simulink model "Model_6DOF"  (R2022a)
settings: Solver=FixedStepAuto  StartTime=0.0  StopTime=Tf  FixedStep=0.05  RelTol=1e-3
values from neighbouring files (symbols this model uses):
  Ba_0 = [0 0 0 0 0 0]    [run.m]
  Bv_0 = [-5.14444 0 0 0 0 0]    [run.m]
  Bx_0 = [0 0 -20 0 0 0]    [run.m]
  psi_ref = 0    [run.m]
  Seastate = 0    [run.m]
  Tf = 5000    [run.m]
  v_ref = Bv_0(1)    [run.m]
  z_ref = Bx_0(3)    [run.m]
undefined symbols (not defined in the file or in its folder): Bb, Cp, Cp_prime, dA_BP1, dA_BP2, dA_Hull, dA_PH, dA_Sail, dA_SProot, dA_X1a, dA_X1b, dA_X2a, dA_X2b, dA_X3a, dA_X3b, dA_X4a, dA_X4b, Ixx, Ixy, Ixz, Iyy, Iyz, Izz, Mb, n_BP1, n_BP2, n_Hull, n_PH, n_Sail, n_SProot, n_X2a, n_X2b, n_X3a, n_X4a, n_X4b, nt_BP1, nt_BP2, nt_Hull, nt_PH, nt_Sail, nt_SProot, nt_X1a, nt_X1b, nt_X2a, nt_X2b, nt_X3a, nt_X3b, nt_X4a, nt_X4b, tknots, vt1_BP1, vt1_BP2, vt1_Hull, vt1_PH, vt1_Sail, vt1_SProot, vt1_X1a, vt1_X1b, vt1_X2a, vt1_X2b ... (+39)
libraries: simulink x8
(part 3 of 5)

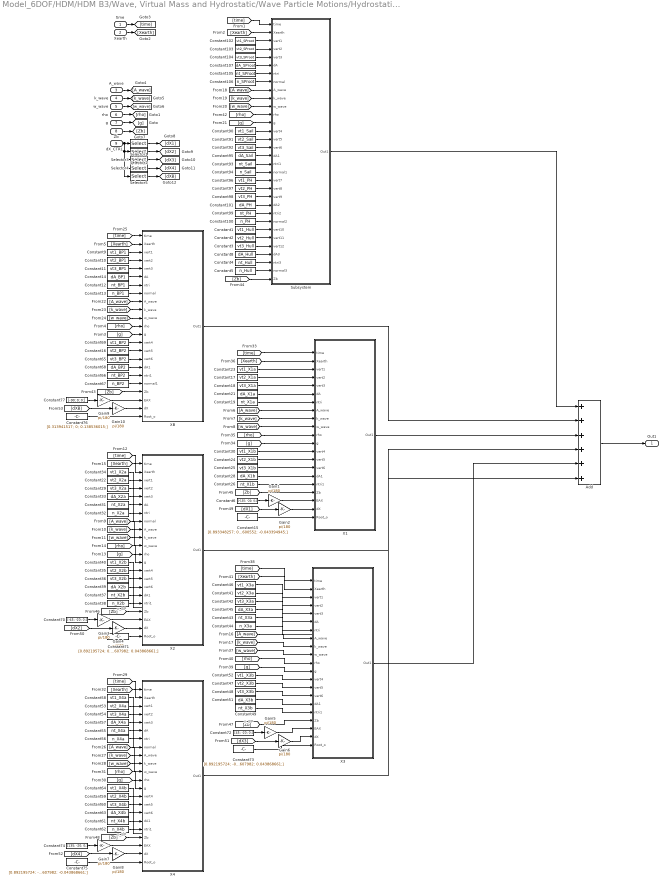
== system Model_6DOF/HDM/HDM B3/Wave, Virtual Mass and Hydrostatic/Wave Particle Motions/Hydrostatic Forces and Moments ==
  note: n_BP
  note: n_BP
  note: n_BP
  time : Inport
  Xearth : Inport  Port=2
  A_wave : Inport  Port=3
  k_wave : Inport  Port=4
  w_wave : Inport  Port=5
  rho : Inport  Port=6
  g : Inport  Port=7
  Zb : Inport  Port=8
  dX_CTRL : Inport  Port=9
  Add : Sum  Inputs=6
  Constant1 : Constant  Value=vt1_Hull
  Constant10 : Constant  Value=vt2_BP1
  Constant100 : Constant  Value=n_PH
  Constant101 : Constant  Value=dA_PH
  Constant102 : Constant  Value=vt1_SProot
  Constant103 : Constant  Value=vt2_SProot
  Constant104 : Constant  Value=vt3_SProot
  Constant105 : Constant  Value=nt_SProot
  Constant106 : Constant  Value=n_SProot
  Constant107 : Constant  Value=dA_SProot
  Constant11 : Constant  Value=vt3_BP1
  Constant12 : Constant  Value=nt_BP1
  Constant13 : Constant  Value=n_BP1
  Constant14 : Constant  Value=dA_BP1
  Constant15 : Constant  Value=|
      | [0.893348257;
      | 0.043600552;
      | -0.043394945;]
  Constant16 : Constant  Value=vt2_BP2
  Constant17 : Constant  Value=vt2_X1a
  Constant18 : Constant  Value=vt3_X1a
  Constant19 : Constant  Value=nt_X1a
  Constant2 : Constant  Value=vt2_Hull
  Constant21 : Constant  Value=dA_X1a
  Constant22 : Constant  Value=vt2_X2a
  Constant23 : Constant  Value=vt1_X1a
  Constant24 : Constant  Value=vt2_X1b
  Constant25 : Constant  Value=vt3_X1b
  Constant26 : Constant  Value=nt_X1b
  Constant28 : Constant  Value=dA_X1b
  Constant29 : Constant  Value=vt3_X2a
  Constant3 : Constant  Value=vt3_Hull
  Constant30 : Constant  Value=vt1_X1b
  Constant31 : Constant  Value=nt_X2a
  Constant32 : Constant  Value=n_X2a
  Constant33 : Constant  Value=dA_X2a
  Constant34 : Constant  Value=vt1_X2a
  Constant35 : Constant  Value=vt2_X2b
  Constant36 : Constant  Value=vt3_X2b
  Constant37 : Constant  Value=nt_X2b
  Constant38 : Constant  Value=n_X2b
  Constant39 : Constant  Value=dA_X2b
  Constant4 : Constant  Value=nt_Hull
  Constant40 : Constant  Value=vt1_X2b
  Constant41 : Constant  Value=vt2_X3a
  Constant42 : Constant  Value=vt3_X3a
  Constant43 : Constant  Value=nt_X3a
  Constant44 : Constant  Value=n_X3a
  Constant45 : Constant  Value=dA_X3a
  Constant46 : Constant  Value=vt1_X3a
  Constant47 : Constant  Value=vt2_X3b
  Constant48 : Constant  Value=vt3_X3b
  Constant49 : Constant  Value=nt_X3b
  Constant5 : Constant  Value=n_Hull
  Constant51 : Constant  Value=dA_X3b
  Constant52 : Constant  Value=vt1_X3b
  Constant53 : Constant  Value=vt2_X4a
  Constant54 : Constant  Value=vt3_X4a
  Constant55 : Constant  Value=nt_X4a
  Constant56 : Constant  Value=n_X4a
  Constant57 : Constant  Value=dA_X4a
  Constant58 : Constant  Value=vt1_X4a
  Constant59 : Constant  Value=vt2_X4b
  Constant6 : Constant  Value=[-135; -20; 0;]
  Constant60 : Constant  Value=vt3_X4b
  Constant61 : Constant  Value=nt_X4b
  Constant62 : Constant  Value=n_X4b
  Constant63 : Constant  Value=dA_X4b
  Constant64 : Constant  Value=vt1_X4b
  Constant65 : Constant  Value=vt3_BP2
  Constant66 : Constant  Value=nt_BP2
  Constant67 : Constant  Value=n_BP2
  Constant68 : Constant  Value=dA_BP2
  Constant69 : Constant  Value=vt1_BP2
  Constant70 : Constant  Value=[-45; -20; 0;]
  Constant71 : Constant  Value=|
      | [0.892195724;
      | 0.043607982;
      | 0.043868661;]
  Constant72 : Constant  Value=[45; -20; 0;]
  Constant73 : Constant  Value=|
      | [0.892195724;
      | -0.043607982;
      | 0.043868661;]
  Constant74 : Constant  Value=[135; -20; 0;]
  Constant75 : Constant  Value=|
      | [0.892195724;
      | -0.043607982;
      | -0.043868661;]
  Constant76 : Constant  Value=|
      | [0.313941517;
      | 0;
      | 0.138536015;]
  Constant77 : Constant  Value=[-90; 0; 0;]
  Constant8 : Constant  Value=dA_Hull
  Constant9 : Constant  Value=vt1_BP1
  Constant90 : Constant  Value=vt1_Sail
  Constant91 : Constant  Value=vt2_Sail
  Constant92 : Constant  Value=vt3_Sail
  Constant93 : Constant  Value=nt_Sail
  Constant94 : Constant  Value=n_Sail
  Constant95 : Constant  Value=dA_Sail
  Constant96 : Constant  Value=vt1_PH
  Constant97 : Constant  Value=vt2_PH
  Constant98 : Constant  Value=vt3_PH
  Constant99 : Constant  Value=nt_PH
  Gain{1..10} (10 alike) : Gain  Gain=pi/180
  Selector1 : Selector  InputPortWidth=5  IndexOptions=Index vector (dialog)  Indices=1  OutputSizes=1
  Selector2 : Selector  InputPortWidth=5  IndexOptions=Index vector (dialog)  Indices=2  OutputSizes=1
  Selector3 : Selector  InputPortWidth=5  IndexOptions=Index vector (dialog)  Indices=3  OutputSizes=1
  Selector4 : Selector  InputPortWidth=5  IndexOptions=Index vector (dialog)  Indices=4  OutputSizes=1
  Selector5 : Selector  InputPortWidth=5  IndexOptions=Index vector (dialog)  Indices=5  OutputSizes=1
  Subsystem : Subsystem
  X1 : Subsystem
  X2 : Subsystem
  X3 : Subsystem
  X4 : Subsystem
  XB : Subsystem
  Out1 : Outport
  wires:
  time/1 -> [time]
  Xearth/1 -> [Xearth]
  A_wave/1 -> [A_wave]
  k_wave/1 -> [k_wave]
  w_wave/1 -> [w_wave]
  rho/1 -> [rho]
  g/1 -> [g]
  Constant94/1 -> Subsystem/19(normal1)
  Constant61/1 -> X4/18(ntri1)
  Constant57/1 -> X4/6(dA)
  [Zb] -> X4/19(Zb)
  [Zb] -> X3/18(Zb)
  Constant101/1 -> Subsystem/23(dA2)
  Constant16/1 -> XB/15(vert5)
  [Zb] -> X1/18(Zb)
  [Zb] -> X2/19(Zb)
  Constant98/1 -> Subsystem/22(vert9)
  Constant99/1 -> Subsystem/24(ntri2)
  Constant37/1 -> X2/18(ntri1)
  [Zb] -> XB/20(Zb)
  [time] -> X3/1(time)
  [Xearth] -> X1/2(Xearth)
  [w_wave] -> Subsystem/11(w_wave)
  Constant93/1 -> Subsystem/18(ntri1)
  [g] -> X2/13(g)
  Constant28/1 -> X1/16(dA1)
  [w_wave] -> X3/10(w_wave)
  Constant8/1 -> Subsystem/29(dA3)
  Constant95/1 -> Subsystem/17(dA1)
  [A_wave] -> X4/9(A_wave)
  Constant33/1 -> X2/6(dA)
  [rho] -> X4/12(rho)
  [time] -> Subsystem/1(time)
  Constant48/1 -> X3/15(vert6)
  [rho] -> Subsystem/12(rho)
  Constant60/1 -> X4/16(vert6)
  [k_wave] -> Subsystem/10(k_wave)
  Constant19/1 -> X1/7(ntri)
  [g] -> Subsystem/13(g)
  Constant102/1 -> Subsystem/3(vert1)
  Constant106/1 -> Subsystem/8(normal)
  [Xearth] -> Subsystem/2(Xearth)
  Constant107/1 -> Subsystem/6(dA)
  Constant105/1 -> Subsystem/7(ntri)
  [g] -> X4/13(g)
  Constant11/1 -> XB/5(vert3)
  Constant34/1 -> X2/3(vert1)
  Constant63/1 -> X4/17(dA1)
  [A_wave] -> X1/8(A_wave)
  Constant41/1 -> X3/4(vert2)
  [k_wave] -> X2/10(k_wave)
  Constant22/1 -> X2/4(vert2)
  Constant49/1 -> X3/17(ntri1)
  [Xearth] -> XB/2(Xearth)
  [rho] -> X2/12(rho)
  [rho] -> X3/11(rho)
  Constant55/1 -> X4/7(ntri)
  Constant45/1 -> X3/6(dA)
  Constant40/1 -> X2/14(vert4)
  Constant18/1 -> X1/5(vert3)
  [g] -> X1/12(g)
  Constant35/1 -> X2/15(vert5)
  Constant39/1 -> X2/17(dA1)
  Constant32/1 -> X2/8(normal)
  Constant47/1 -> X3/14(vert5)
  [w_wave] -> X4/11(w_wave)
  Constant44/1 -> ?
  [k_wave] -> X1/9(k_wave)
  Constant53/1 -> X4/4(vert2)
  [w_wave] -> XB/11(w_wave)
  [Xearth] -> X2/2(Xearth)
  [time] -> XB/1(time)
  [rho] -> XB/12(rho)
  Constant4/1 -> Subsystem/30(ntri3)
  Constant59/1 -> X4/15(vert5)
  Constant51/1 -> X3/16(dA1)
  Constant52/1 -> X3/13(vert4)
  Constant14/1 -> XB/6(dA)
  [Xearth] -> X3/2(Xearth)
  Constant25/1 -> X1/15(vert6)
  Constant67/1 -> XB/19(normal1)
  [Zb] -> Subsystem/32(Zb)
  Constant65/1 -> XB/16(vert6)
  Constant104/1 -> Subsystem/5(vert3)
  Constant13/1 -> XB/8(normal)
  Constant69/1 -> XB/14(vert4)
  Constant43/1 -> X3/7(ntri)
  [k_wave] -> X3/9(k_wave)
  [A_wave] -> X2/9(A_wave)
  Constant17/1 -> X1/4(vert2)
  [k_wave] -> XB/10(k_wave)
  Constant68/1 -> XB/17(dA1)
  Constant46/1 -> X3/3(vert1)
  Constant23/1 -> X1/3(vert1)
  Constant9/1 -> XB/3(vert1)
  Constant62/1 -> ?
  [A_wave] -> XB/9(A_wave)
  Constant26/1 -> X1/17(ntri1)
  Constant56/1 -> X4/8(normal)
  Constant24/1 -> X1/14(vert5)
  Constant12/1 -> XB/7(ntri)
  [g] -> X3/12(g)
  [w_wave] -> X1/10(w_wave)
  Constant100/1 -> Subsystem/25(normal2)
  Constant92/1 -> Subsystem/16(vert6)
  Constant30/1 -> X1/13(vert4)
  [time] -> X2/1(time)
  [rho] -> X1/11(rho)
  Constant91/1 -> Subsystem/15(vert5)
  [time] -> X1/1(time)
  Constant1/1 -> Subsystem/26(vert10)
  Constant31/1 -> X2/7(ntri)
  [w_wave] -> X2/11(w_wave)
  Constant21/1 -> X1/6(dA)
  Constant90/1 -> Subsystem/14(vert4)
  Constant96/1 -> Subsystem/20(vert7)
  Constant36/1 -> X2/16(vert6)
  Constant29/1 -> X2/5(vert3)
  [Xearth] -> X4/2(Xearth)
  Constant64/1 -> X4/14(vert4)
  Constant97/1 -> Subsystem/21(vert8)
  Constant2/1 -> Subsystem/27(vert11)
  Constant66/1 -> XB/18(ntri1)
  Constant54/1 -> X4/5(vert3)
  Constant38/1 -> ?
  [k_wave] -> X4/10(k_wave)
  [time] -> X4/1(time)
  Constant10/1 -> XB/4(vert2)
  [A_wave] -> Subsystem/9(A_wave)
  Add/1 -> Out1/1
  Constant103/1 -> Subsystem/4(vert2)
  Constant3/1 -> Subsystem/28(vert12)
  [g] -> XB/13(g)
  Constant42/1 -> X3/5(vert3)
  Constant58/1 -> X4/3(vert1)
  Constant5/1 -> Subsystem/31(normal3)
  [A_wave] -> X3/8(A_wave)
  Zb/1 -> [Zb]
  Constant6/1 -> Gain1/1
  Gain1/1 -> X1/19(EAX)
  dX_CTRL/1 -> Selector2/1, Selector3/1, Selector5/1, Selector4/1, Selector1/1
  Selector1/1 -> [dX1]
  Selector2/1 -> [dX2]
  Selector3/1 -> [dX3]
  Selector4/1 -> [dX4]
  Selector5/1 -> [dXB]
  [dX1] -> Gain2/1
  Gain2/1 -> X1/20(dX)
  Constant15/1 -> X1/21(Root_o)
  Constant70/1 -> Gain3/1
  Gain3/1 -> X2/20(EAX)
  [dX2] -> Gain4/1
  Gain4/1 -> X2/21(dX)
  Constant71/1 -> X2/22(Root_o)
  Gain5/1 -> X3/19(EAX)
  [dX3] -> Gain6/1
  Constant72/1 -> Gain5/1
  Gain6/1 -> X3/20(dX)
  Constant73/1 -> X3/21(Root_o)
  Constant75/1 -> X4/22(Root_o)
  Gain7/1 -> X4/20(EAX)
  Constant74/1 -> Gain7/1
  [dX4] -> Gain8/1
  Gain8/1 -> X4/21(dX)
  Constant77/1 -> Gain9/1
  Gain9/1 -> XB/21(EAX)
  [dXB] -> Gain10/1
  Constant76/1 -> XB/23(Root_o)
  Gain10/1 -> XB/22(dX)
  X4/1(Out1) -> Add/6
  X3/1(Out1) -> Add/5
  X2/1(Out1) -> Add/4
  X1/1(Out1) -> Add/3
  XB/1(Out1) -> Add/2
  Subsystem/1(Out1) -> Add/1

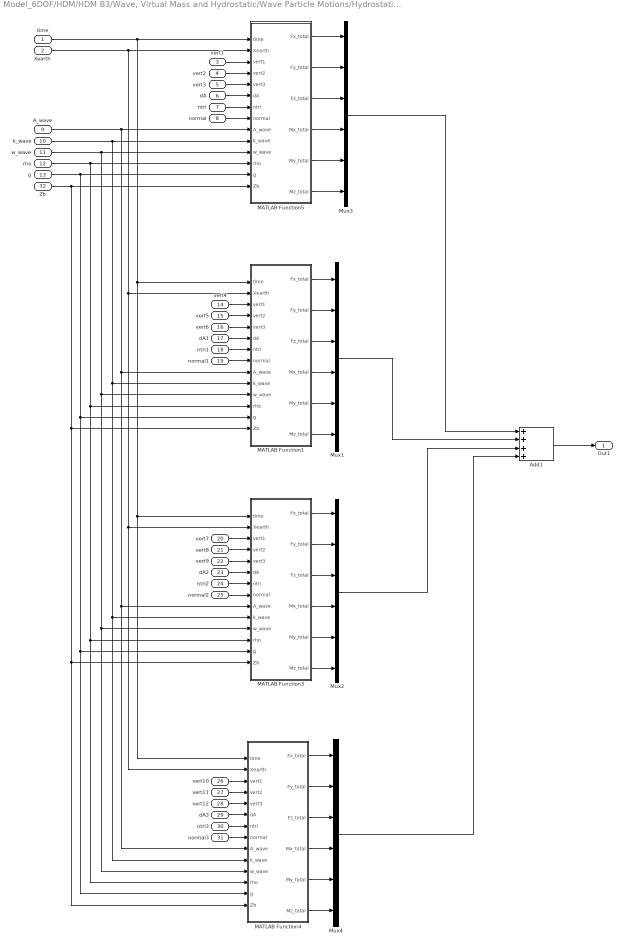
== system Model_6DOF/HDM/HDM B3/Wave, Virtual Mass and Hydrostatic/Wave Particle Motions/Hydrostatic Forces and Moments/Subsystem ==
  time : Inport
  Xearth : Inport  Port=2
  vert1 : Inport  Port=3
  vert2 : Inport  Port=4
  vert3 : Inport  Port=5
  dA : Inport  Port=6
  ntri : Inport  Port=7
  normal : Inport  Port=8
  A_wave : Inport  Port=9
  k_wave : Inport  Port=10
  w_wave : Inport  Port=11
  rho : Inport  Port=12
  g : Inport  Port=13
  vert4 : Inport  Port=14
  vert5 : Inport  Port=15
  vert6 : Inport  Port=16
  dA1 : Inport  Port=17
  ntri1 : Inport  Port=18
  normal1 : Inport  Port=19
  vert7 : Inport  Port=20
  vert8 : Inport  Port=21
  vert9 : Inport  Port=22
  dA2 : Inport  Port=23
  ntri2 : Inport  Port=24
  normal2 : Inport  Port=25
  vert10 : Inport  Port=26
  vert11 : Inport  Port=27
  vert12 : Inport  Port=28
  dA3 : Inport  Port=29
  ntri3 : Inport  Port=30
  normal3 : Inport  Port=31
  Zb : Inport  Port=32
  Add1 : Sum  Inputs=4
  MATLAB Function1 : MATLAB Function  TreatAsAtomicUnit=on
  MATLAB Function3 : MATLAB Function  TreatAsAtomicUnit=on
  MATLAB Function4 : MATLAB Function  TreatAsAtomicUnit=on
  MATLAB Function5 : MATLAB Function  TreatAsAtomicUnit=on
  Mux{1..4} (4 alike) : Mux  Inputs=6
  Out1 : Outport
  wires:
  ntri1/1 -> MATLAB Function1/7(ntri)
  rho/1 -> MATLAB Function5/12(rho), MATLAB Function1/12(rho), MATLAB Function4/12(rho), MATLAB Function3/12(rho)
  vert5/1 -> MATLAB Function1/4(vert2)
  MATLAB Function5/5(My_total) -> Mux3/5
  time/1 -> MATLAB Function5/1(time), MATLAB Function1/1(time), MATLAB Function4/1(time), MATLAB Function3/1(time)
  Xearth/1 -> MATLAB Function5/2(Xearth), MATLAB Function4/2(Xearth), MATLAB Function3/2(Xearth), MATLAB Function1/2(Xearth)
  vert7/1 -> MATLAB Function3/3(vert1)
  MATLAB Function5/4(Mx_total) -> Mux3/4
  Mux3/1 -> Add1/1
  normal1/1 -> MATLAB Function1/8(normal)
  A_wave/1 -> MATLAB Function5/9(A_wave), MATLAB Function1/9(A_wave), MATLAB Function4/9(A_wave), MATLAB Function3/9(A_wave)
  MATLAB Function5/3(Fz_total) -> Mux3/3
  k_wave/1 -> MATLAB Function5/10(k_wave), MATLAB Function1/10(k_wave), MATLAB Function4/10(k_wave), MATLAB Function3/10(k_wave)
  w_wave/1 -> MATLAB Function5/11(w_wave), MATLAB Function1/11(w_wave), MATLAB Function4/11(w_wave), MATLAB Function3/11(w_wave)
  MATLAB Function5/2(Fy_total) -> Mux3/2
  ntri/1 -> MATLAB Function5/7(ntri)
  g/1 -> MATLAB Function5/13(g), MATLAB Function1/13(g), MATLAB Function4/13(g), MATLAB Function3/13(g)
  dA2/1 -> MATLAB Function3/6(dA)
  MATLAB Function5/1(Fx_total) -> Mux3/1
  vert12/1 -> MATLAB Function4/5(vert3)
  normal3/1 -> MATLAB Function4/8(normal)
  vert4/1 -> MATLAB Function1/3(vert1)
  vert9/1 -> MATLAB Function3/5(vert3)
  normal/1 -> MATLAB Function5/8(normal)
  dA/1 -> MATLAB Function5/6(dA)
  MATLAB Function5/6(Mz_total) -> Mux3/6
  vert11/1 -> MATLAB Function4/4(vert2)
  ntri2/1 -> MATLAB Function3/7(ntri)
  ntri3/1 -> MATLAB Function4/7(ntri)
  dA3/1 -> MATLAB Function4/6(dA)
  vert2/1 -> MATLAB Function5/4(vert2)
  Add1/1 -> Out1/1
  vert6/1 -> MATLAB Function1/5(vert3)
  vert3/1 -> MATLAB Function5/5(vert3)
  normal2/1 -> MATLAB Function3/8(normal)
  dA1/1 -> MATLAB Function1/6(dA)
  vert10/1 -> MATLAB Function4/3(vert1)
  vert1/1 -> MATLAB Function5/3(vert1)
  vert8/1 -> MATLAB Function3/4(vert2)
  Zb/1 -> MATLAB Function5/14(Zb), MATLAB Function1/14(Zb), MATLAB Function3/14(Zb), MATLAB Function4/14(Zb)
  Mux2/1 -> Add1/3
  MATLAB Function1/6(Mz_total) -> Mux1/6
  Mux1/1 -> Add1/2
  MATLAB Function1/1(Fx_total) -> Mux1/1
  MATLAB Function1/2(Fy_total) -> Mux1/2
  MATLAB Function1/3(Fz_total) -> Mux1/3
  MATLAB Function1/4(Mx_total) -> Mux1/4
  MATLAB Function1/5(My_total) -> Mux1/5
  MATLAB Function3/5(My_total) -> Mux2/5
  MATLAB Function3/4(Mx_total) -> Mux2/4
  MATLAB Function3/3(Fz_total) -> Mux2/3
  MATLAB Function3/2(Fy_total) -> Mux2/2
  MATLAB Function3/1(Fx_total) -> Mux2/1
  MATLAB Function3/6(Mz_total) -> Mux2/6
  MATLAB Function4/6(Mz_total) -> Mux4/6
  MATLAB Function4/1(Fx_total) -> Mux4/1
  MATLAB Function4/2(Fy_total) -> Mux4/2
  MATLAB Function4/3(Fz_total) -> Mux4/3
  MATLAB Function4/4(Mx_total) -> Mux4/4
  MATLAB Function4/5(My_total) -> Mux4/5
  Mux4/1 -> Add1/4

== system Model_6DOF/HDM/HDM B3/Wave, Virtual Mass and Hydrostatic/Wave Particle Motions/Hydrostatic Forces and Moments/X1 ==
  time : Inport
  Xearth : Inport  Port=2
  vert1 : Inport  Port=3
  vert2 : Inport  Port=4
  vert3 : Inport  Port=5
  dA : Inport  Port=6
  ntri : Inport  Port=7
  A_wave : Inport  Port=8
  k_wave : Inport  Port=9
  w_wave : Inport  Port=10
  rho : Inport  Port=11
  g : Inport  Port=12
  vert4 : Inport  Port=13
  vert5 : Inport  Port=14
  vert6 : Inport  Port=15
  dA1 : Inport  Port=16
  ntri1 : Inport  Port=17
  Zb : Inport  Port=18
  EAX : Inport  Port=19
  dX : Inport  Port=20
  Root_o : Inport  Port=21
  Add1 : Sum
  CG : Constant  Value=[32.3114; 0; 0;]
  MATLAB Function1 : MATLAB Function  TreatAsAtomicUnit=on
  MATLAB Function4 : MATLAB Function  TreatAsAtomicUnit=on
  Mux1 : Mux  Inputs=6
  Mux2 : Mux  Inputs=6
  Out1 : Outport
  wires:
  ntri1/1 -> MATLAB Function1/7(ntri)
  dA1/1 -> MATLAB Function1/6(dA)
  vert6/1 -> MATLAB Function1/5(vert3)
  vert5/1 -> MATLAB Function1/4(vert2)
  vert4/1 -> MATLAB Function1/3(vert1)
  Zb/1 -> MATLAB Function1/13(Zb), MATLAB Function4/13(Zb)
  vert2/1 -> MATLAB Function4/4(vert2)
  ntri/1 -> MATLAB Function4/7(ntri)
  time/1 -> MATLAB Function4/1(time), MATLAB Function1/1(time)
  vert1/1 -> MATLAB Function4/3(vert1)
  Mux1/1 -> Add1/2
  vert3/1 -> MATLAB Function4/5(vert3)
  Mux2/1 -> Add1/1
  MATLAB Function4/2(Fy_total) -> Mux2/2
  MATLAB Function4/6(Mz_total) -> Mux2/6
  g/1 -> MATLAB Function1/12(g), MATLAB Function4/12(g)
  k_wave/1 -> MATLAB Function4/9(k_wave), MATLAB Function1/9(k_wave)
  dA/1 -> MATLAB Function4/6(dA)
  MATLAB Function4/5(My_total) -> Mux2/5
  MATLAB Function1/3(Fz_total) -> Mux1/3
  Add1/1 -> Out1/1
  MATLAB Function1/1(Fx_total) -> Mux1/1
  MATLAB Function4/1(Fx_total) -> Mux2/1
  MATLAB Function1/4(Mx_total) -> Mux1/4
  A_wave/1 -> MATLAB Function1/8(A_wave), MATLAB Function4/8(A_wave)
  rho/1 -> MATLAB Function1/11(rho), MATLAB Function4/11(rho)
  Xearth/1 -> MATLAB Function4/2(Xearth), MATLAB Function1/2(Xearth)
  MATLAB Function1/2(Fy_total) -> Mux1/2
  w_wave/1 -> MATLAB Function1/10(w_wave), MATLAB Function4/10(w_wave)
  MATLAB Function4/4(Mx_total) -> Mux2/4
  MATLAB Function4/3(Fz_total) -> Mux2/3
  EAX/1 -> MATLAB Function1/14(EAX), MATLAB Function4/14(EAX)
  dX/1 -> MATLAB Function4/15(dX), MATLAB Function1/15(dX)
  Root_o/1 -> MATLAB Function1/16(origin), MATLAB Function4/16(origin)
  CG/1 -> MATLAB Function1/17(xcg), MATLAB Function4/17(xcg)
  MATLAB Function1/5(My_total) -> Mux1/5
  MATLAB Function1/6(Mz_total) -> Mux1/6

== system Model_6DOF/HDM/HDM B3/Wave, Virtual Mass and Hydrostatic/Wave Particle Motions/Hydrostatic Forces and Moments/X2 ==
  time : Inport
  Xearth : Inport  Port=2
  vert1 : Inport  Port=3
  vert2 : Inport  Port=4
  vert3 : Inport  Port=5
  dA : Inport  Port=6
  ntri : Inport  Port=7
  normal : Inport  Port=8
  A_wave : Inport  Port=9
  k_wave : Inport  Port=10
  w_wave : Inport  Port=11
  rho : Inport  Port=12
  g : Inport  Port=13
  vert4 : Inport  Port=14
  vert5 : Inport  Port=15
  vert6 : Inport  Port=16
  dA1 : Inport  Port=17
  ntri1 : Inport  Port=18
  Zb : Inport  Port=19
  EAX : Inport  Port=20
  dX : Inport  Port=21
  Root_o : Inport  Port=22
  Add1 : Sum
  CG : Constant  Value=[32.3114; 0; 0;]
  MATLAB Function1 : MATLAB Function  TreatAsAtomicUnit=on
  MATLAB Function4 : MATLAB Function  TreatAsAtomicUnit=on
  Mux1 : Mux  Inputs=6
  Mux2 : Mux  Inputs=6
  Out1 : Outport
  wires:
  MATLAB Function1/6(Mz_total) -> Mux1/6
  MATLAB Function1/5(My_total) -> Mux1/5
  CG/1 -> MATLAB Function1/17(xcg), MATLAB Function4/17(xcg)
  Root_o/1 -> MATLAB Function1/16(origin), MATLAB Function4/16(origin)
  dX/1 -> MATLAB Function1/15(dX), MATLAB Function4/15(dX)
  EAX/1 -> MATLAB Function1/14(EAX), MATLAB Function4/14(EAX)
  MATLAB Function4/3(Fz_total) -> Mux2/3
  MATLAB Function4/4(Mx_total) -> Mux2/4
  w_wave/1 -> MATLAB Function1/10(w_wave), MATLAB Function4/10(w_wave)
  MATLAB Function1/2(Fy_total) -> Mux1/2
  Xearth/1 -> MATLAB Function1/2(Xearth), MATLAB Function4/2(Xearth)
  rho/1 -> MATLAB Function1/11(rho), MATLAB Function4/11(rho)
  A_wave/1 -> MATLAB Function1/8(A_wave), MATLAB Function4/8(A_wave)
  MATLAB Function1/4(Mx_total) -> Mux1/4
  MATLAB Function4/1(Fx_total) -> Mux2/1
  MATLAB Function1/1(Fx_total) -> Mux1/1
  Add1/1 -> Out1/1
  MATLAB Function1/3(Fz_total) -> Mux1/3
  MATLAB Function4/5(My_total) -> Mux2/5
  dA/1 -> MATLAB Function4/6(dA)
  k_wave/1 -> MATLAB Function1/9(k_wave), MATLAB Function4/9(k_wave)
  g/1 -> MATLAB Function1/12(g), MATLAB Function4/12(g)
  MATLAB Function4/6(Mz_total) -> Mux2/6
  MATLAB Function4/2(Fy_total) -> Mux2/2
  Mux2/1 -> Add1/1
  vert3/1 -> MATLAB Function4/5(vert3)
  Mux1/1 -> Add1/2
  vert1/1 -> MATLAB Function4/3(vert1)
  time/1 -> MATLAB Function1/1(time), MATLAB Function4/1(time)
  normal/1 -> ?
  ntri/1 -> MATLAB Function4/7(ntri)
  vert2/1 -> MATLAB Function4/4(vert2)
  Zb/1 -> MATLAB Function1/13(Zb), MATLAB Function4/13(Zb)
  vert4/1 -> MATLAB Function1/3(vert1)
  vert5/1 -> MATLAB Function1/4(vert2)
  vert6/1 -> MATLAB Function1/5(vert3)
  dA1/1 -> MATLAB Function1/6(dA)
  ntri1/1 -> MATLAB Function1/7(ntri)

== system Model_6DOF/HDM/HDM B3/Wave, Virtual Mass and Hydrostatic/Wave Particle Motions/Hydrostatic Forces and Moments/X3 ==
  time : Inport
  Xearth : Inport  Port=2
  vert1 : Inport  Port=3
  vert2 : Inport  Port=4
  vert3 : Inport  Port=5
  dA : Inport  Port=6
  ntri : Inport  Port=7
  A_wave : Inport  Port=8
  k_wave : Inport  Port=9
  w_wave : Inport  Port=10
  rho : Inport  Port=11
  g : Inport  Port=12
  vert4 : Inport  Port=13
  vert5 : Inport  Port=14
  vert6 : Inport  Port=15
  dA1 : Inport  Port=16
  ntri1 : Inport  Port=17
  Zb : Inport  Port=18
  EAX : Inport  Port=19
  dX : Inport  Port=20
  Root_o : Inport  Port=21
  Add1 : Sum
  CG : Constant  Value=[32.3114; 0; 0;]
  MATLAB Function1 : MATLAB Function  TreatAsAtomicUnit=on
  MATLAB Function4 : MATLAB Function  TreatAsAtomicUnit=on
  Mux1 : Mux  Inputs=6
  Mux2 : Mux  Inputs=6
  Out1 : Outport
  wires:
  ntri1/1 -> MATLAB Function1/7(ntri)
  dA1/1 -> MATLAB Function1/6(dA)
  vert6/1 -> MATLAB Function1/5(vert3)
  vert5/1 -> MATLAB Function1/4(vert2)
  vert4/1 -> MATLAB Function1/3(vert1)
  Zb/1 -> MATLAB Function4/13(Zb), MATLAB Function1/13(Zb)
  vert2/1 -> MATLAB Function4/4(vert2)
  ntri/1 -> MATLAB Function4/7(ntri)
  time/1 -> MATLAB Function4/1(time), MATLAB Function1/1(time)
  vert1/1 -> MATLAB Function4/3(vert1)
  Mux1/1 -> Add1/2
  vert3/1 -> MATLAB Function4/5(vert3)
  Mux2/1 -> Add1/1
  MATLAB Function4/2(Fy_total) -> Mux2/2
  MATLAB Function4/6(Mz_total) -> Mux2/6
  g/1 -> MATLAB Function4/12(g), MATLAB Function1/12(g)
  k_wave/1 -> MATLAB Function4/9(k_wave), MATLAB Function1/9(k_wave)
  dA/1 -> MATLAB Function4/6(dA)
  MATLAB Function4/5(My_total) -> Mux2/5
  MATLAB Function1/3(Fz_total) -> Mux1/3
  Add1/1 -> Out1/1
  MATLAB Function1/1(Fx_total) -> Mux1/1
  MATLAB Function4/1(Fx_total) -> Mux2/1
  MATLAB Function1/4(Mx_total) -> Mux1/4
  A_wave/1 -> MATLAB Function4/8(A_wave), MATLAB Function1/8(A_wave)
  rho/1 -> MATLAB Function4/11(rho), MATLAB Function1/11(rho)
  Xearth/1 -> MATLAB Function4/2(Xearth), MATLAB Function1/2(Xearth)
  MATLAB Function1/2(Fy_total) -> Mux1/2
  w_wave/1 -> MATLAB Function4/10(w_wave), MATLAB Function1/10(w_wave)
  MATLAB Function4/4(Mx_total) -> Mux2/4
  MATLAB Function4/3(Fz_total) -> Mux2/3
  EAX/1 -> MATLAB Function4/14(EAX), MATLAB Function1/14(EAX)
  dX/1 -> MATLAB Function4/15(dX), MATLAB Function1/15(dX)
  Root_o/1 -> MATLAB Function4/16(origin), MATLAB Function1/16(origin)
  CG/1 -> MATLAB Function4/17(xcg), MATLAB Function1/17(xcg)
  MATLAB Function1/5(My_total) -> Mux1/5
  MATLAB Function1/6(Mz_total) -> Mux1/6

== system Model_6DOF/HDM/HDM B3/Wave, Virtual Mass and Hydrostatic/Wave Particle Motions/Hydrostatic Forces and Moments/X4 ==
  time : Inport
  Xearth : Inport  Port=2
  vert1 : Inport  Port=3
  vert2 : Inport  Port=4
  vert3 : Inport  Port=5
  dA : Inport  Port=6
  ntri : Inport  Port=7
  normal : Inport  Port=8
  A_wave : Inport  Port=9
  k_wave : Inport  Port=10
  w_wave : Inport  Port=11
  rho : Inport  Port=12
  g : Inport  Port=13
  vert4 : Inport  Port=14
  vert5 : Inport  Port=15
  vert6 : Inport  Port=16
  dA1 : Inport  Port=17
  ntri1 : Inport  Port=18
  Zb : Inport  Port=19
  EAX : Inport  Port=20
  dX : Inport  Port=21
  Root_o : Inport  Port=22
  Add1 : Sum
  CG : Constant  Value=[32.3114; 0; 0;]
  MATLAB Function1 : MATLAB Function  TreatAsAtomicUnit=on
  MATLAB Function4 : MATLAB Function  TreatAsAtomicUnit=on
  Mux1 : Mux  Inputs=6
  Mux2 : Mux  Inputs=6
  Out1 : Outport
  wires:
  MATLAB Function1/6(Mz_total) -> Mux1/6
  MATLAB Function1/5(My_total) -> Mux1/5
  CG/1 -> MATLAB Function1/17(xcg), MATLAB Function4/17(xcg)
  Root_o/1 -> MATLAB Function1/16(origin), MATLAB Function4/16(origin)
  dX/1 -> MATLAB Function1/15(dX), MATLAB Function4/15(dX)
  EAX/1 -> MATLAB Function1/14(EAX), MATLAB Function4/14(EAX)
  MATLAB Function4/3(Fz_total) -> Mux2/3
  MATLAB Function4/4(Mx_total) -> Mux2/4
  w_wave/1 -> MATLAB Function1/10(w_wave), MATLAB Function4/10(w_wave)
  MATLAB Function1/2(Fy_total) -> Mux1/2
  Xearth/1 -> MATLAB Function1/2(Xearth), MATLAB Function4/2(Xearth)
  rho/1 -> MATLAB Function4/11(rho), MATLAB Function1/11(rho)
  A_wave/1 -> MATLAB Function1/8(A_wave), MATLAB Function4/8(A_wave)
  MATLAB Function1/4(Mx_total) -> Mux1/4
  MATLAB Function4/1(Fx_total) -> Mux2/1
  MATLAB Function1/1(Fx_total) -> Mux1/1
  Add1/1 -> Out1/1
  MATLAB Function1/3(Fz_total) -> Mux1/3
  MATLAB Function4/5(My_total) -> Mux2/5
  dA/1 -> MATLAB Function4/6(dA)
  k_wave/1 -> MATLAB Function1/9(k_wave), MATLAB Function4/9(k_wave)
  g/1 -> MATLAB Function1/12(g), MATLAB Function4/12(g)
  MATLAB Function4/6(Mz_total) -> Mux2/6
  MATLAB Function4/2(Fy_total) -> Mux2/2
  Mux2/1 -> Add1/1
  vert3/1 -> MATLAB Function4/5(vert3)
  Mux1/1 -> Add1/2
  vert1/1 -> MATLAB Function4/3(vert1)
  time/1 -> MATLAB Function1/1(time), MATLAB Function4/1(time)
  normal/1 -> ?
  ntri/1 -> MATLAB Function4/7(ntri)
  vert2/1 -> MATLAB Function4/4(vert2)
  Zb/1 -> MATLAB Function1/13(Zb), MATLAB Function4/13(Zb)
  vert4/1 -> MATLAB Function1/3(vert1)
  vert5/1 -> MATLAB Function1/4(vert2)
  vert6/1 -> MATLAB Function1/5(vert3)
  dA1/1 -> MATLAB Function1/6(dA)
  ntri1/1 -> MATLAB Function1/7(ntri)

== system Model_6DOF/HDM/HDM B3/Wave, Virtual Mass and Hydrostatic/Wave Particle Motions/Hydrostatic Forces and Moments/XB ==
  time : Inport
  Xearth : Inport  Port=2
  vert1 : Inport  Port=3
  vert2 : Inport  Port=4
  vert3 : Inport  Port=5
  dA : Inport  Port=6
  ntri : Inport  Port=7
  normal : Inport  Port=8
  A_wave : Inport  Port=9
  k_wave : Inport  Port=10
  w_wave : Inport  Port=11
  rho : Inport  Port=12
  g : Inport  Port=13
  vert4 : Inport  Port=14
  vert5 : Inport  Port=15
  vert6 : Inport  Port=16
  dA1 : Inport  Port=17
  ntri1 : Inport  Port=18
  normal1 : Inport  Port=19
  Zb : Inport  Port=20
  EAX : Inport  Port=21
  dX : Inport  Port=22
  Root_o : Inport  Port=23
  Add1 : Sum
  CG : Constant  Value=[32.3114; 0; 0;]
  MATLAB Function1 : MATLAB Function  TreatAsAtomicUnit=on
  MATLAB Function4 : MATLAB Function  TreatAsAtomicUnit=on
  Mux1 : Mux  Inputs=6
  Mux2 : Mux  Inputs=6
  Out1 : Outport
  wires:
  MATLAB Function1/6(Mz_total) -> Mux1/6
  MATLAB Function1/5(My_total) -> Mux1/5
  CG/1 -> MATLAB Function1/17(xcg), MATLAB Function4/17(xcg)
  Root_o/1 -> MATLAB Function1/16(origin), MATLAB Function4/16(origin)
  dX/1 -> MATLAB Function1/15(dX), MATLAB Function4/15(dX)
  EAX/1 -> MATLAB Function1/14(EAX), MATLAB Function4/14(EAX)
  MATLAB Function4/3(Fz_total) -> Mux2/3
  MATLAB Function4/4(Mx_total) -> Mux2/4
  w_wave/1 -> MATLAB Function1/10(w_wave), MATLAB Function4/10(w_wave)
  MATLAB Function1/2(Fy_total) -> Mux1/2
  Xearth/1 -> MATLAB Function1/2(Xearth), MATLAB Function4/2(Xearth)
  rho/1 -> MATLAB Function1/11(rho), MATLAB Function4/11(rho)
  A_wave/1 -> MATLAB Function1/8(A_wave), MATLAB Function4/8(A_wave)
  MATLAB Function1/4(Mx_total) -> Mux1/4
  MATLAB Function4/1(Fx_total) -> Mux2/1
  MATLAB Function1/1(Fx_total) -> Mux1/1
  Add1/1 -> Out1/1
  MATLAB Function1/3(Fz_total) -> Mux1/3
  MATLAB Function4/5(My_total) -> Mux2/5
  dA/1 -> MATLAB Function4/6(dA)
  k_wave/1 -> MATLAB Function1/9(k_wave), MATLAB Function4/9(k_wave)
  g/1 -> MATLAB Function1/12(g), MATLAB Function4/12(g)
  MATLAB Function4/6(Mz_total) -> Mux2/6
  MATLAB Function4/2(Fy_total) -> Mux2/2
  Mux2/1 -> Add1/1
  vert3/1 -> MATLAB Function4/5(vert3)
  Mux1/1 -> Add1/2
  vert1/1 -> MATLAB Function4/3(vert1)
  time/1 -> MATLAB Function1/1(time), MATLAB Function4/1(time)
  normal/1 -> ?
  ntri/1 -> MATLAB Function4/7(ntri)
  vert2/1 -> MATLAB Function4/4(vert2)
  Zb/1 -> MATLAB Function1/13(Zb), MATLAB Function4/13(Zb)
  vert4/1 -> MATLAB Function1/3(vert1)
  vert5/1 -> MATLAB Function1/4(vert2)
  vert6/1 -> MATLAB Function1/5(vert3)
  dA1/1 -> MATLAB Function1/6(dA)
  ntri1/1 -> MATLAB Function1/7(ntri)
  normal1/1 -> ?

== matlab function Model_6DOF/Controller/pf_controller ==
  settings: updateMethod=DISCRETE
  data: v_ref input; z_ref input; psi_ref input; Bv input; Bx input; dX output; Ts parameter; n output
function [dX,n]   = fcn(v_ref,z_ref,psi_ref,Bv,Bx,Ts)

persistent zerr_prev zerr_int_prev thetaerr_prev thetaerr_int_prev psierr_prev psierr_int_prev

%% Initialize
if isempty(zerr_prev)
        zerr_prev = 0;
        zerr_int_prev = 0;
        thetaerr_prev = 0;
        thetaerr_int_prev = 0;
        psierr_prev = 0;
        psierr_int_prev = 0;
end


%% Variables for feedback
x = Bx(1); y = Bx(2); z = Bx(3); phi = Bx(4); theta = Bx(5); psi = Bx(6);
p = [x;y;z];
uN = Bv(1); vN = Bv(2); wN = Bv(3); pB = Bv(4); qB=Bv(5); rB = Bv(6);
uB = -uN; vB = -vN; wB = wN;


%% Gains
KP_APz = 3;
KI_APz = 0.1044;
KD_APz = 3;

KP_APtheta = 3;
KI_APtheta = 0.1466;
KD_APtheta = 3;

KP_APpsi = 3;
KI_APpsi = 0;
KD_APpsi = 12.199;

speed_cmd = -5;
KP_n = 5;
FF_inv = 4;






%% Autopilot (depth)
zerr = z_ref - z;
zerrint = zerr*Ts+zerr_int_prev;
zerrdot = (zerr-zerr_prev)/Ts;
dvz = KP_APz*zerr+KI_APz*zerrint+KD_APz*zerrdot;

theta_ref = 0;
thetaerr = (theta_ref - theta)*180/pi;
thetaerrint = thetaerr*Ts+thetaerr_int_prev;
thetaerrdot = (thetaerr-thetaerr_prev)/Ts;
dvtheta = KP_APtheta*thetaerr+KI_APtheta*thetaerrint+KD_APtheta*thetaerrdot;

dv = dvz + dvtheta;

%% Autopilot (yaw)
psierr = (psi_ref - psi)*180/pi;
psierrint = psierr*Ts+psierr_int_prev;
psierrdot = (psierr-psierr_prev)/Ts;
dh = KP_APpsi*psierr+KI_APpsi*psierrint+KD_APpsi*psierrdot;


%% Control Allocation
d1 = -dv+dh; 
d2 = -dv-dh; 
d3 = dv-dh; 
d4 = dv+dh; 
d5 = dv; 
dX = [d1 ; d2 ; d3 ; d4 ; d5];


%% Prop
n = -v_ref/FF_inv;


%% Save variables for next loop
zerr_prev = zerr;
zerr_int_prev = zerrint;
thetaerr_prev = thetaerr;
thetaerr_int_prev = thetaerrint;
psierr_prev = psierr;
psierr_int_prev = psierrint;

== matlab function Model_6DOF/Controller/pf_controller2 ==
  settings: updateMethod=DISCRETE
  data: Bv input; Bx input; dX output; ref input; n output; Cp parameter; Cp_prime parameter; stop output; adap input; pd output; pddot output; tknots parameter; Tf parameter
function [dX,n,stop,pd,pddot]   = fcn(Bv,Bx,ref,Cp,Cp_prime,adap, tknots, Tf)
%pd,NomegaNI,

%% Declare variables for integration and differentiation
Ts = 0.05; % Time step
stop = 0;
persistent gamma gammadot xuq xdq xur xdr RDT_prev RTI_prev ... 
    qerr_prev qerr_int_prev rerr_prev rerr_int_prev




%% Variables for feedback
x = Bx(1); y = Bx(2); z = Bx(3); phi = Bx(4); theta = Bx(5); psi = Bx(6);
p = [x;y;z];
uN = Bv(1); vN = Bv(2); wN = Bv(3); pB = Bv(4); qB=Bv(5); rB = Bv(6);
speed_cmd = ref;
uB = -uN; vB = -vN; wB = wN;

%% Control Parameters  
% Gains and parameters for PF
vcmd = 5; 
kgamma = 1; 
kR = 0.1; 
d = 250; 

% Gains for PF augmentation
Tsq = Ts; Tsr = Ts;
Amq = -0.1; Bmq = 0.25; Cmq = 0.4; 
Phiinvq = 50.1251; Lambdaq = 0.4;
Aoq = [-0.0496   -0.5024    0.5251; 1.3605   -0.5493    1.2008; -1.0756    0.8116   -1.5010]; 
Boq = [0.1240 ; -0.6198 ; 0.7748]; 
Coq = [0 0.8 0.64];
Amr = -0.1; Bmr = 0.25; Cmr = 0.4; 
Phiinvr = 50.1251; Lambdar = 0.4;
Aor = [-0.0300 -0.0192 -0.0082; 0.0156 0 0; 0 0.0078 0]; 
Bor = [0.25 ; 0 ; 0]; 
Cor = [0 0 0.1311];


% Autopilot Gain
KP_APq = 30*10^2;
KI_APq = 0*50*10^0;
KD_APq = 0;
KP_APr = 30*10^2;
KI_APr = 0*50*10^0;
KD_APr = 0;
% Speed controller gain
KP_n = 5;
FF_inv = 4;




%% Initialize
if isempty(gamma)
        gamma = 0; gammadot = 1;
        xuq = zeros(length(Aoq),1);
        xdq = Cmq'*inv(Cmq*Cmq')*qB;
        xur = zeros(length(Aor),1);
        xdr = Cmr'*inv(Cmr*Cmr')*rB;
        RDT_prev = zeros(3);
        RTI_prev = zeros(3);
        qerr_prev = 0;
        qerr_int_prev = 0;
        rerr_prev = 0;
        rerr_int_prev = 0;
        segment = 0;
end




%% Compute Rotation Matrices
alpha = -atan2(wB,sqrt(uB^2+vB^2));
beta = atan2(vB,uB);

RBW = [cos(alpha)*cos(beta) cos(alpha)*sin(beta) -sin(alpha);...
       -sin(beta)            cos(beta)             0;...
       cos(beta)*sin(alpha) sin(alpha)*sin(beta)  cos(alpha)];
   
RWB = RBW';


RNI = [ cos(psi)*cos(theta), cos(psi)*sin(phi)*sin(theta) - cos(phi)*sin(psi), sin(phi)*sin(psi) + cos(phi)*cos(psi)*sin(theta);
        cos(theta)*sin(psi), cos(phi)*cos(psi) + sin(phi)*sin(psi)*sin(theta), cos(phi)*sin(psi)*sin(theta) - cos(psi)*sin(phi);
         -sin(theta),                              cos(theta)*sin(phi),                              cos(phi)*cos(theta)];
     
RBN = [-1 0 0; 0 -1 0; 0 0 1];

RWI = RNI*RBN*RBW';

RWN = RBN*RWB;
RNW = RWN';



%pd = PiecewiseBernsteinPoly(Cp, tknots, gamma);
pd = BernsteinPoly(Cp, gamma, 0, Tf);
%pd_prime = PiecewiseBernsteinPoly(Cp_prime, tknots, gamma);
pd_prime = BernsteinPoly(Cp_prime, gamma, 0, Tf);
pddot = pd_prime*gammadot;
if gamma >= Tf
    stop = 1;
end


t1hat = pd_prime/norm(pd_prime);
t2hat = [-pd_prime(2) ; pd_prime(1) ; 0 ]/norm([-pd_prime(2) ; pd_prime(1) ; 0 ]);
t3hat = cross(t1hat,t2hat);

RTI = [t1hat' ; t2hat' ; t3hat']';
RIT = RTI';







%% Compute gamma
gammadot = max(0.0001,((sqrt(uN^2+vN^2+wN^2)*RWI*[1;0;0] + kgamma*(p-pd))'*RTI*[1;0;0])/norm(pd_prime));
gamma = gamma + gammadot*Ts;







%% Compute desired angular rate
pT = RIT*(p-pd); %path following error

yT = pT(2); zT = pT(3);
toterr_y = yT; toterr_z = zT;
b1D = [d/(sqrt(d^2+toterr_y^2+toterr_z^2)) ; -toterr_y/(sqrt(d^2+toterr_y^2+toterr_z^2)) ; -toterr_z/(sqrt(d^2+toterr_y^2+toterr_z^2))];
b2D = [toterr_y/(sqrt(d^2+toterr_y^2)) ; d/(sqrt(d^2+toterr_y^2)) ; 0];
b3D = cross(b1D,b2D);
RDT = [b1D b2D b3D]; % Desired frame
% RTD = eye(3);
RTD = RDT';

Rtilde = RDT'*RIT*RWI;

eR = 0.5*[Rtilde(1,3); -Rtilde(1,2)];
PiR = [0 1 0 ; 0 0 1];


RDTdot = (RDT-RDT_prev)./Ts;
RTIdot = (RTI-RTI_prev)./Ts;

SDomegaDT = RTD*RDTdot;
DomegaDT = [-SDomegaDT(2,3); SDomegaDT(1,3) ; -SDomegaDT(1,2)];
STomegaTI = RIT*RTIdot;
TomegaTI = [-STomegaTI(2,3); STomegaTI(1,3) ; -STomegaTI(1,2)];

qc = [0 1 0]*Rtilde'*(RTD*TomegaTI + DomegaDT) - [1 0]*2*kR*eR;
rc = [0 0 1]*Rtilde'*(RTD*TomegaTI + DomegaDT) - [0 1]*2*kR*eR;


RNWdot = zeros(3,3);
SNomegaNW = RNW'*RNWdot;
NomegaNW = [-SNomegaNW(2,3) ; SNomegaNW(1,3); -SNomegaNW(1,2)];
NomegaNI = NomegaNW + RWN*[0;qc;rc];

q_ref = [0 1 0]*NomegaNI;
r_ref = [0 0 1]*NomegaNI;


RIW = RWI';
b1 = RWI(:,1);






%% L1 Augmentation - dive

if adap 

    ydq = Cmq*xdq;

    sigmaq = -Phiinvq*expm(Lambdaq*(Amq/Lambdaq)*Tsq)*1*(ydq-qB);

    xuq_next = expm(Aoq*Tsq)*xuq + inv(Aoq)*(expm(Aoq*Tsq)-eye(3))*(Boq*expm(-Amq*Tsq)*sigmaq);
    Kgq = -inv(Cmq*inv(Amq)*Bmq);
    udq = Kgq*q_ref - Coq*xuq;

    xdq_next = expm(Amq*Tsq)*xdq + inv(Amq)*(expm(Amq*Tsq)-eye(length(Amq)))*(Bmq*udq + sigmaq);

    qaug = udq;

else 

    qaug = q_ref;

    xdq_next = xdq;
    xuq_next = xuq;

end



%% Autopilot

qerr = qaug - qB;
qerrint = qerr*Ts+qerr_int_prev;
qerrdot = (qerr-qerr_prev)/Ts;
dv = KP_APq*qerr+KI_APq*qerrint+KD_APq*qerrdot;


%% L1 Augmentation - steering
if adap
    ydr = Cmr*xdr;

    sigmar = -Phiinvr*expm(Lambdar*(Amr/Lambdar)*Tsr)*1*(ydr-rB);

    xur_next = expm(Aor*Tsr)*xur + inv(Aor)*(expm(Aor*Tsr)-eye(3))*(Bor*expm(-Amr*Tsr)*sigmar);
    Kgr = -inv(Cmr*inv(Amr)*Bmr);
    udr = Kgr*r_ref - Cor*xur;

    xdr_next = expm(Amr*Tsr)*xdr + inv(Amr)*(expm(Amr*Tsr)-eye(length(Amr)))*(Bmr*udr + sigmar);

    raug = udr;

else 

    raug = r_ref;

    xdr_next = xdr;
    xur_next = xur;

end




%% Autopilot
rerr = raug - rB;
rerrint = rerr*Ts+rerr_int_prev;
rerrdot = (rerr-rerr_prev)/Ts;
dh = KP_APr*rerr+KI_APr*rerrint+KD_APr*rerrdot;



%% Control Allocation
d1 = -dv+dh; 
d2 = -dv-dh; 
d3 = dv-dh; 
d4 = dv+dh; 
d5 = dv; 

dX = [d1 ; d2 ; d3 ; d4 ; d5];






%% Speed Controller
% if x > -2500
%     s_d = ref;
% else
%     s_d = ref-.1/400*(x+2500);
% end
% n = -(s_d/FF_inv + KP_n*(s_d-uN));
%n = -(speed_cmd/FF_inv + KP_n*(speed_cmd-uN));
%speed_cmd = ref*min(1,.7*exp(-(gamma-400)/350)+.3);
n = -speed_cmd/FF_inv;



% gammaout = gamma;
% gammadotout = gammadot;
% pdes = pd;


%% Save variables for next loop
xuq = xuq_next;
xdq = xdq_next;
xur = xur_next;
xdr = xdr_next;
RDT_prev = RDT;
RTI_prev = RTI;
qerr_prev = qerr;
qerr_int_prev = qerrint;
rerr_prev = rerr;
rerr_int_prev = rerrint;


%% Functions requried for Bernstein Polynomials

function  poly_t  = PiecewiseBernsteinPoly(Cp,tknots,time)

% INPUTS:
% 
% OUTPUT:
% 
% 
% Written by: Venanzio Cichella       

%%%%%%%%%%%%%%%%%%%%%%%%%%%%%%%%%%%%%%%%%%%%%%

M = length(tknots)-1;
[dim, totN] = size(Cp);
N = totN/M - 1;

poly_t = zeros(dim,length(time));

for i = 1 : M
    for k = 1 : length(time)   
        if time(k) >= tknots(i) && time(k) <= tknots(i+1) 
            t = time(k);
            if i < M
                poly_t(:,k) = BernsteinPoly(Cp(:,(i-1)*N+i:i*N+i),t,tknots(i),tknots(i+1));
            else
                poly_t(:,k) = BernsteinPoly(Cp(:,(i-1)*N+i:end),t,tknots(i),tknots(i+1));
            end
        end
    end
end







function  poly_t  = BernsteinPoly(Cp,t,t0,tf)

% INPUTS:
% Cp is a matrix n by N+1 (n: dimension of polynomial, N: order of polynomial) 
% t is a time vector
% OUTPUT:
% poly_t: n-dimensional polynomial evaluated at each time t

% if t is a scalar, it returns the value of Bernstein Poly at t in [t0,tf]
% if t0 and tf are not provided, it returns the value of Bernstein Poly at t in [0,1]

% Written by: Venanzio Cichella       

%%%%%%%%%%%%%%%%%%%%%%%%%%%%%%%%%%%%%%%%%%%%%%



[~, N] = size(Cp);
N = N-1;

% if length(t) > 1
%     B = BernsteinMatrix_a2b(N,t)';
%     poly_t = Cp*B;
% else
%     if ~exist('t0','var')
%         B = BernsteinMatrix_a2b(N,t)';
%         poly_t = Cp*B;
%     else
%         B = BernsteinMatrix_a2b(N,t,t0,tf)';
%         poly_t = Cp*B;
%     end
% end
B = BernsteinMatrix_a2b(N,t,t0,tf)';
poly_t = Cp*B;






function  poly_t  = BernsteinPolyStable(Cp,t)

[m,n] = size(Cp);
poly_t = zeros(m,length(t));
count = 0;
for i = 1 : length(t)
    [~,poly_t(:,i)] = deCasteljau(Cp,t(i));
    count = count + 1;
end




function [Cpout, Pos] = deCasteljau(Cp,lambda)          
% Cpout are the control points of two curves.
% i.e.    cptsPA = Cpout(:, 1:length(Cp(1,:)));
%         cptsPB = Cpout(:, length(Cp(1,:)):end);
% Pos is the position at lambda
% lambda must be in [0,1]

[m,n] = size(Cp);
n = n-1;

A = (1-lambda)*eye(n,n);
B = lambda*eye(n,n);
C = zeros(n+1,n);

C(1:n,:) = C(1:n,:) + A; 
C(2:n+1,:) = C(2:n+1,:) + B;

Cpout = zeros(m,(n+1)+n);

Cptemp = Cp;
Cp1 = zeros(m,n);
Cp2 = zeros(m,n);

for i = n:-1:1
    Cptemp(:,1:i) = Cptemp(:,1:i+1)*C(1:i+1,1:i);
    Cp1(:,n+1-i) = Cptemp(:,1);
    Cp2(:,i) = Cptemp(:,i);
end

Cpout = [Cp(:,1) Cp1 Cp2(:,2:end) Cp(:,end)];
Pos = Cp1(:,end);





function b = BernsteinMatrix_a2b(N, t, tmin, tmax)

% Inputs: order N, time vector t = [t0 ... tm], no need for tmin and tmax.
% Output: b = [b0N(t0) b1N(t0) ... bNN(t0);
%              b0N(t1) b1N(t1) ... bNN(t1);
%              ...
%              b0N(tm) b1N(tm) ... bNN(tm);
% Use: If Cp is a row vector of N+1 control points,
%       the Nth order Bezier curve is given by xN=Cp*b';
% This function is used in BernsteinPoly

% Alternatively
% Inputs: order n, scalar time t', tmin and tmax
% Output: b = [b0n(t') b1n(t') ... bnn(t')]
% Use: If Cp is a row vector of N+1 control points,
%       the Nth order Bezier curve evaluated at t' is given by xn=Cp*b';
% Comment: This is more efficient but not as robust as de Casteljau
%           It works best for low-order curves

% Written by: Venanzio Cichella       

%%%%%%%%%%%%%%%%%%%%%%%%%%%%%%%%%%%%%%%%%%%%%%

if length(t) > 1
    tmax = t(length(t));
    tmin = t(1);
end

% if ~exist('tmin','var')
%     tmin = 0; tmax = 1;
% end



% compute B(j+1) = binomial(n, j), j = 0..n
t = t';
B = ones(N+1, 1); 
for j = 1:ceil(N/2)
  B(j+1) = B(j)*(N+1-j)/j;
  B(N+1-j) = B(j+1);
end
% compute T(i, j) = (t(i)-tmin)^j, TT(i, j) = (tmax-t(i))^(N-j)
T = ones(length(t), N+1);
TT = ones(length(t), N+1);
% turn a row t into a column t so that 
% we can do diag(t)*T(:,j) by t.*T(:,j)
tp = reshape(t, length(t), 1)-tmin;
ttp = tmax - t;
% Compute binomial(N, j)*(t(i)-tmin)^j*(tmax-t(i))^(N-j)
for j = 1:N 
  T(:, j+1) = tp .* T(:, j); 
  T(:, j) = T(:, j) .* B(j);
 TT(:,N+1-j) = ttp .* TT(:,N+2-j);
end

% Compute binomial(N, j)*(t(i)-tmin)^j*(tmax-t(i))^(N-j)/((tmax-tmin)^N)
b =  T.*TT./((tmax-tmin)^N);






function xN = LagrangePoly(x,tnodes,time)

%% Get polynomials
n = length(x);

basis_polynomials = cell(n,1); %basis polynomials for values t

for i = 1:n
    basis_polynomials{i} = 0;
    numerator = 1;
    denominator = 1;
    for k = 1:n
        if i~=k
            numerator = numerator.*(time-tnodes(k));
            denominator = denominator.*(tnodes(i)-tnodes(k));
        end
    end
    basis_polynomials{i} = numerator./denominator;
end


% then find the Lagrange polynomial coefficients
xN = 0;

for k = 1:n
    xN = xN + x(k)*basis_polynomials{k};
end

== matlab function Model_6DOF/HDM/HDM B3/Wave, Virtual Mass and Hydrostatic/Wave Particle Motions/Hydrostatic Forces and Moments/XB/MATLAB Function1 ==
  data: time input; Xearth input; Fx_total output; vert1 input; vert2 input; vert3 input; dA input; ntri input; A_wave input; k_wave input; w_wave input; rho input; g input; Fy_total output; Fz_total output; Mx_total output; My_total output; Mz_total output; Zb input; EAX input; dX input; origin input; xcg input
function [Fx_total,Fy_total,Fz_total,Mx_total,My_total,Mz_total]= fcn(time,Xearth,vert1,vert2,vert3,dA,ntri,A_wave,k_wave,w_wave,rho,g,Zb,EAX,dX,origin,xcg)
%EAX=Appendage eulater angle in local coordinate
%its=number of time steps to skip writing grid

x_e=Xearth(1); y_e=Xearth(2); z_e=Xearth(3);
phi=Xearth(4); theta=Xearth(5); psi=Xearth(6);
phiX=EAX(1); thetaX=EAX(2); psiX=EAX(3);


RMat=[cos(theta)*cos(psi) -cos(phi)*sin(psi)+sin(phi)*sin(theta)*cos(psi)  sin(phi)*sin(psi)+cos(phi)*sin(theta)*cos(psi); ...
      cos(theta)*sin(psi)  cos(phi)*cos(psi)+sin(phi)*sin(theta)*sin(psi) -sin(phi)*cos(psi)+cos(phi)*sin(theta)*sin(psi); ...
     -sin(theta)                             sin(phi)*cos(theta)                             cos(phi)*cos(theta)];  
RMATX=[cos(thetaX)*cos(psiX) -cos(phiX)*sin(psiX)+sin(phiX)*sin(thetaX)*cos(psiX)  sin(phiX)*sin(psiX)+cos(phiX)*sin(thetaX)*cos(psiX); ...
      cos(thetaX)*sin(psiX)  cos(phiX)*cos(psiX)+sin(phiX)*sin(thetaX)*sin(psiX) -sin(phiX)*cos(psiX)+cos(phiX)*sin(thetaX)*sin(psiX); ...
     -sin(thetaX)                             sin(phiX)*cos(thetaX)                             cos(phiX)*cos(thetaX)];  
RMATD=[cos(0)*cos(dX) -cos(0)*sin(dX)+sin(0)*sin(0)*cos(dX)  sin(0)*sin(dX)+cos(0)*sin(0)*cos(dX); ...
      cos(0)*sin(dX)  cos(0)*cos(dX)+sin(0)*sin(0)*sin(dX) -sin(0)*cos(dX)+cos(0)*sin(0)*sin(dX); ...
     -sin(0)                             sin(0)*cos(0)                             cos(0)*cos(0)];  


%Rotating the vertices to put in ship coordinate
for i=1:ntri 
    V1=[vert1(i,1); vert1(i,2); vert1(i,3);];
    V2=[vert2(i,1); vert2(i,2); vert2(i,3);];
    V3=[vert3(i,1); vert3(i,2); vert3(i,3);];
        
    %rotating to local z coordinate
    V1_o=inv(RMATX)*(V1-origin*70.2+xcg);
    V2_o=inv(RMATX)*(V2-origin*70.2+xcg);
    V3_o=inv(RMATX)*(V3-origin*70.2+xcg);
    
    %rotating for corresponding appendage deflection
    V1_x=RMATD*V1_o;
    V2_x=RMATD*V2_o;
    V3_x=RMATD*V3_o;
    
        %re-positioning the appendage to local vectors
    V1_r=RMATX*V1_x;
    V2_r=RMATX*V2_x;
    V3_r=RMATX*V3_x;
    
    %re-assigning vertices
    
    for j=1:3
    vert1(i,j)=V1_r(j)+origin(j)*70.2-xcg(j);
    vert2(i,j)=V2_r(j)+origin(j)*70.2-xcg(j);
    vert3(i,j)=V3_r(j)+origin(j)*70.2-xcg(j);
    end  
end

 
%position of mid points in earth coordinate;
mp1=zeros(ntri,3);
mp2=zeros(ntri,3);
mp3=zeros(ntri,3);
nA =zeros(ntri,3);

P1=zeros(ntri,1);
P2=zeros(ntri,1);
P3=zeros(ntri,1);

%position vector of mid points from the CG
r1=zeros(ntri,3);
r2=zeros(ntri,3);
r3=zeros(ntri,3);

v1_w=zeros(ntri,3);
v2_w=zeros(ntri,3);
v3_w=zeros(ntri,3);
n_w=zeros(ntri,3);

%Area of triangle, product of area and unit normal, position vector to each mid-point

for i=1:ntri
    %Area of each triangle
    A=[vert2(i,1)-vert1(i,1); vert2(i,2)-vert1(i,2); vert2(i,3)-vert1(i,3);];
    B=[vert3(i,1)-vert1(i,1); vert3(i,2)-vert1(i,2); vert3(i,3)-vert1(i,3);];
    n=cross(A,B)/norm(cross(A,B));
    C=[n(1); n(2); n(3);];
    %C=[normal(i,1); normal(i,2); normal(i,3);];

    
    %A*n vector calculation
    for j=1:3
        nA(i,j)=dA(i).*C(j);    
    end
    
    %position vector to each mid point of each edge
    for j=1:3
        r1(i,j)=0.5*(vert1(i,j)+vert2(i,j));
        r2(i,j)=0.5*(vert1(i,j)+vert3(i,j));
        r3(i,j)=0.5*(vert2(i,j)+vert3(i,j));
    end
end

%computing mid point location between vertices in earth coordinate
for i=1:ntri
    MP1=RMat*[r1(i,1); r1(i,2); r1(i,3);]+[x_e; y_e; z_e;];
    MP2=RMat*[r2(i,1); r2(i,2); r2(i,3);]+[x_e; y_e; z_e;];
    MP3=RMat*[r3(i,1); r3(i,2); r3(i,3);]+[x_e; y_e; z_e;];
    
    v1i=RMat*[vert1(i,1); vert1(i,2); vert1(i,3);]+[x_e; y_e; z_e;];
    v2i=RMat*[vert2(i,1); vert2(i,2); vert2(i,3);]+[x_e; y_e; z_e;];
    v3i=RMat*[vert3(i,1); vert3(i,2); vert3(i,3);]+[x_e; y_e; z_e;];
    
    for j=1:3
        v1_w(i,j)=v1i(j); v2_w(i,j)=v2i(j); v3_w(i,j)=v3i(j);
        mp1(i,j)=MP1(j);  mp2(i,j)=MP2(j);  mp3(i,j)=MP3(j);
    end
end

for i=1:ntri
    A=[v2_w(i,1)-v1_w(i,1); v2_w(i,2)-v1_w(i,2); v2_w(i,3)-v1_w(i,3);];
    B=[v3_w(i,1)-v1_w(i,1); v3_w(i,2)-v1_w(i,2); v3_w(i,3)-v1_w(i,3);];
    n=cross(A,B)/norm(cross(A,B));
    dA(i,1)=0.5*norm(cross(A,B));
    n_w(i,1)=n(1); n_w(i,2)=n(2); n_w(i,3)=n(3);
end



%computing forces and moments for each triangle
Fx_total=0; Fy_total=0; Fz_total=0;
Mx_total=0; My_total=0; Mz_total=0;

for i=1:ntri
    p1=-rho*g*(mp1(i,3)-A_wave*exp(k_wave.*mp1(i,3)).*sin(k_wave*mp1(i,1)-w_wave.*time));
    p2=-rho*g*(mp2(i,3)-A_wave*exp(k_wave.*mp2(i,3)).*sin(k_wave*mp2(i,1)-w_wave.*time));
    p3=-rho*g*(mp3(i,3)-A_wave*exp(k_wave.*mp3(i,3)).*sin(k_wave*mp3(i,1)-w_wave.*time));
    
    dFx=-nA(i,1)*(p1+p2+p3)./3;
    dFy=-nA(i,2)*(p1+p2+p3)./3;
    dFz=-nA(i,3)*(p1+p2+p3)./3;
    
    dP =-p1.*[r1(i,1); r1(i,2); r1(i,3)-Zb;]...
        -p2.*[r2(i,1); r2(i,2); r2(i,3)-Zb;]...
        -p3.*[r3(i,1); r3(i,2); r3(i,3)-Zb;];
    N =[nA(i,1); nA(i,2); nA(i,3);];
    dM=cross(dP,N);
    Fx_total=Fx_total+dFx;
    Fy_total=Fy_total+dFy;
    Fz_total=Fz_total+dFz;
    Mx_total=Mx_total+dM(1)/3;
    My_total=My_total+dM(2)/3;
    Mz_total=Mz_total+dM(3)/3;
end
end

== matlab function Model_6DOF/HDM/Integration and Coord. Transfrom/Coordinate Transform/MATLAB Function2 ==
  data: Bx input; out output; Bv input
function out = fcn(Bx,Bv)
u = Bv(1); v = Bv(2); w = Bv(3); p = Bv(4); q = Bv(5); r = Bv(6);
x = Bx(1); y = Bx(2); z = Bx(3); phi = Bx(4); theta = Bx(5); psi = Bx(6);

Vx_ship=[u; v; w];
Vr_ship=[p; q; r];

RMat=[cos(theta)*cos(psi) -cos(phi)*sin(psi)+sin(phi)*sin(theta)*cos(psi)  sin(phi)*sin(psi)+cos(phi)*sin(theta)*cos(psi); ...
      cos(theta)*sin(psi)  cos(phi)*cos(psi)+sin(phi)*sin(theta)*sin(psi) -sin(phi)*cos(psi)+cos(phi)*sin(theta)*sin(psi); ...
              -sin(theta)                             sin(phi)*cos(theta)                             cos(phi)*cos(theta)];

QMat=[1  tan(theta)*sin(phi) tan(theta)*cos(phi); ...
      0  cos(phi)           -sin(phi); ...
      0  sin(phi)/cos(theta) cos(phi)/cos(theta)];
   
Vx_earth=RMat*Vx_ship;
Vr_earth=QMat*Vr_ship;


out = [Vx_earth(1); Vx_earth(2); Vx_earth(3); Vr_earth(1); Vr_earth(2); Vr_earth(3)];
